simulink library "LopesDevelopmentLibrary"  (R2015b)
settings: Solver=ode45  StartTime=0.0  StopTime=10.0  RelTol=1e-3
values from neighbouring files (symbols this model uses):
  d2r = @(d) d*(pi/180)    [LopesDevelopmentLibrary_LoadParameters.m]
  ts = LopesParams.ts    [LopesDevelopmentLibrary_LoadParameters.m]
undefined symbols (not defined in the file or in its folder): anyParameterChanged, DiscIntNeverNeededParam, gcbh, LAP, LHF, LKF, LopesParams, macaddr, mxpcnetworkconfig, mxpcrtudprx, mxpcrtudptx, patientParametersChanged, port, PX, PZ, RAP, RHF, RKF, SelectorLOPESInSize, StrideTime_s, Time
undefined symbols (not defined in the file): LopesParamsSendDataArrayLen
libraries: LopesDevelopmentLibrary x327, simulink x100, dspmtrx3 x49, xpciplib x6, xpcnetworkbufferlib x5, dspsigops x4, dspstat3 x3, xpcethernetlib x2, visionstatistics x2, xpcseriallib x2, LopesDevelopmentLibraryTest x1, nmc x1
(part 7 of 12)

== system LopesDevelopmentLibrary/GaitPhaseDetection/Gait Phase Detection with Wrapper/No speed detection ==
  note: If COP is 5x closer to foot 1 than foot 2, foot 2 is assumed to be in swing
  note: Detection
      | 1 = stance phase
      | 2 = swing phase
  note: If the treadmill velocity is above 0.05 and 250 ms have passed
      | since the start of the simulation, gait initiation can be detected using the "normal" method
      | If Velocity of treadmill is too low, the COP is used to estimate swing/stance
  curVel : Inport
  CartesianPositions : Inport  Port=2
  Treadmill : Inport  Port=3
  "   " : MinMax
  "        " : simulink/Discrete/Tapped Delay  vinit=0  samptime=-1  NumDelays=250  DelayOrder=Oldest  includeCurrent=off
  Ankle_L_XZ : Selector  InputPortWidth=21  IndexOptions=Index vector (dialog)  Indices=[10 12]  OutputSizes=1
  Ankle_R_XZ : Selector  InputPortWidth=21  IndexOptions=Index vector (dialog)  Indices=[19 21]  OutputSizes=1
  COP_XZ : Selector  InputPortWidth=7  IndexOptions=Index vector (dialog)  Indices=[5 6]  OutputSizes=1
  Compare To Constant : simulink/Logic and Bit Operations/Compare To Constant  relop=<=  const=0.2  OutDataTypeStr=boolean
  Compare To Constant1 : simulink/Logic and Bit Operations/Compare To Constant  relop=>=  const=0.05  OutDataTypeStr=uint8  ZeroCross=off
  Compare To Constant2 : simulink/Logic and Bit Operations/Compare To Constant  relop=<=  const=0.2  OutDataTypeStr=boolean
  Constant : Constant  Value=2
  Constant1 : Constant
  Data Type Conversion : DataTypeConversion
  DistLeft : Fcn  Expr=((u(1) - u(3))^2 + (u(2) - u(4))^2)^0.5
  DistRight : Fcn  Expr=((u(1) - u(3))^2 + (u(2) - u(4))^2)^0.5
  Divide : Product  Inputs=*/
  Divide1 : Product  Inputs=*/
  LeftFoot : Switch  Criteria=u2 > Threshold
  Mux : Mux  Inputs=2
  Mux1 : Mux  Inputs=2
  RightFoot : Switch  Criteria=u2 > Threshold
  gaitSwitch : Outport
  Left : Outport  Port=2
  Right : Outport  Port=3
  wires:
  RightFoot/1 -> Right/1
  LeftFoot/1 -> Left/1
  Constant1/1 -> LeftFoot/3, RightFoot/3
  Constant/1 -> RightFoot/1, LeftFoot/1
  Compare To Constant2/1 -> LeftFoot/2
  Compare To Constant/1 -> RightFoot/2
  Divide1/1 -> Compare To Constant2/1
  Divide/1 -> Compare To Constant/1
  DistRight/1 -> Divide1/1, Divide/2
  DistLeft/1 -> Divide/1, Divide1/2
  Mux1/1 -> DistRight/1
  Ankle_R_XZ/1 -> Mux1/1
  COP_XZ/1 -> Mux/2, Mux1/2
  Ankle_L_XZ/1 -> Mux/1
  Mux/1 -> DistLeft/1
  Treadmill/1 -> COP_XZ/1
  CartesianPositions/1 -> Ankle_L_XZ/1, Ankle_R_XZ/1
  "   "/1 -> Compare To Constant1/1
  "        "/1 -> "   "/1
  Data Type Conversion/1 -> gaitSwitch/1
  curVel/1 -> "        "/1
  Compare To Constant1/1 -> Data Type Conversion/1

== system LopesDevelopmentLibrary/GaitPhaseDetection/Gait Phase Detection with Wrapper/Phase_selection ==
  LeftWalking : Inport
  RightWalking : Inport  Port=2
  Gait_switch : Inport  Port=3
  ankle_x_l : Inport  Port=4
  ankle_x_r : Inport  Port=5
  LeftStop : Inport  Port=6
  RightStop : Inport  Port=7
  Delay : Delay  DelayLength=1  InitialCondition=0
  MATLAB Function : MATLAB Function  TreatAsAtomicUnit=on
  Phase : Outport
  wires:
  RightStop/1 -> MATLAB Function/4(rightStop)
  LeftStop/1 -> MATLAB Function/3(leftStop)
  ankle_x_r/1 -> MATLAB Function/7(right_x)
  ankle_x_l/1 -> MATLAB Function/6(left_x)
  Gait_switch/1 -> MATLAB Function/5(switchSignal)
  RightWalking/1 -> MATLAB Function/2(rightWalking)
  LeftWalking/1 -> MATLAB Function/1(leftWalking)
  Delay/1 -> MATLAB Function/8(prev)
  MATLAB Function/1(y) -> Phase/1, Delay/1

== system LopesDevelopmentLibrary/GaitPhaseDetection/Gait Phase Detection with Wrapper/RightLegWalking ==
  note: Right foot detection
      | 1 = stance phase
      | 2 = swing phase
  ankle_y_r_dot : Inport
  ankle_x_r_dot : Inport  Port=2
  knee_angle_dot : Inport  Port=3
  belt_speed : Inport  Port=4
  Add2 : Sum  OutDataTypeStr=double
  Heel strike detection : Subsystem
  Heel strike_safety : Subsystem
  Logical Operator2 : Logic  Operator=OR  AllPortsSameDT=off  OutDataTypeStr=boolean
  Sample and Hold2 : dspsigops/Sample and Hold  trig=Rising edge  initCond=1  latchinput=off
  Toe-off detection : Subsystem
  right : Outport  OutDataTypeStr=double
  wires:
  knee_angle_dot/1 -> Toe-off detection/2(knee_angle_dot)
  Heel strike_safety/1(Heel_strike_safety) -> Logical Operator2/2
  belt_speed/1 -> Heel strike_safety/2(belt_speed)
  Toe-off detection/1(Toe_off) -> Add2/2
  Heel strike detection/1(Heel_strike) -> Logical Operator2/1
  ankle_y_r_dot/1 -> Heel strike detection/1(ankle_y_dot)  "ankle_y_dot"
  ankle_x_r_dot/1 -> Toe-off detection/1(ankle_x_dot), Heel strike detection/2(ankle_x_dot), Heel strike_safety/1(ankle_x_dot)  "ankle_x_dot"
  Add2/1 -> Sample and Hold2/1, Sample and Hold2/Trigger
  Logical Operator2/1 -> Add2/1
  Sample and Hold2/1 -> right/1

== system LopesDevelopmentLibrary/GaitPhaseDetection/Gait Phase Detection with Wrapper/Smart derivative ==
  note: The filter order is regulated by the belt speed to promote
      | efficiency and accuracy
  ankle_y_l : Inport
  ankle_x_l : Inport  Port=2
  angle_knee_l : Inport  Port=3
  ankle_y_r : Inport  Port=4
  ankle_x_r : Inport  Port=5
  angle_knee_r : Inport  Port=6
  treadmill speed : Inport  Port=7
  Filtered derivative : Subsystem
  Filtered derivative1 : Subsystem
  Filtered derivative2 : Subsystem
  Filtered derivative3 : Subsystem
  Filtered derivative4 : Subsystem
  Filtered derivative5 : Subsystem
  belt_speed to cut-off : Subsystem
  ankle_y_l_dot : Outport
  ankle_x_l_dot : Outport  Port=2
  angle_knee_l_dot : Outport  Port=3
  ankle_y_r_dot : Outport  Port=4
  ankle_x_r_dot : Outport  Port=5
  angle_knee_r_dot : Outport  Port=6
  wires:
  Filtered derivative1/1(x_dot) -> ankle_x_l_dot/1
  treadmill speed/1 -> belt_speed to cut-off/1(belt speed)
  belt_speed to cut-off/1(cut-off (hz)) -> Filtered derivative/2(cut-off (hz)), Filtered derivative1/2(cut-off (hz)), Filtered derivative2/2(cut-off (hz)), Filtered derivative3/2(cut-off (hz)), Filtered derivative4/2(cut-off (hz)), Filtered derivative5/2(cut-off (hz))
  Filtered derivative5/1(x_dot) -> angle_knee_r_dot/1
  Filtered derivative4/1(x_dot) -> ankle_x_r_dot/1
  Filtered derivative3/1(x_dot) -> ankle_y_r_dot/1
  Filtered derivative2/1(x_dot) -> angle_knee_l_dot/1
  angle_knee_r/1 -> Filtered derivative5/1(x)
  ankle_x_r/1 -> Filtered derivative4/1(x)
  ankle_y_r/1 -> Filtered derivative3/1(x)
  angle_knee_l/1 -> Filtered derivative2/1(x)
  ankle_x_l/1 -> Filtered derivative1/1(x)
  Filtered derivative/1(x_dot) -> ankle_y_l_dot/1
  ankle_y_l/1 -> Filtered derivative/1(x)

== system LopesDevelopmentLibrary/GaitPhaseDetection/Gait Phase detection/Data selection ==
  Cart_pos : Inport
  Treadmill : Inport  Port=2
  Angle_l : Subsystem
  Angle_r : Subsystem
  Selector : Selector  InputPortWidth=21  IndexOptions=Index vector (dialog)  Indices=[11]  OutputSizes=1
  Selector1 : Selector  InputPortWidth=21  IndexOptions=Index vector (dialog)  Indices=[20]  OutputSizes=1
  Selector10 : Selector  InputPortWidth=21  IndexOptions=Index vector (dialog)  Indices=[16 17 18]  OutputSizes=1
  Selector11 : Selector  InputPortWidth=21  IndexOptions=Index vector (dialog)  Indices=[13 14 15]  OutputSizes=1
  Selector2 : Selector  InputPortWidth=21  IndexOptions=Index vector (dialog)  Indices=[19]  OutputSizes=1
  Selector3 : Selector  InputPortWidth=21  IndexOptions=Index vector (dialog)  Indices=[10]  OutputSizes=1
  Selector4 : Selector  InputPortWidth=7  IndexOptions=Index vector (dialog)  Indices=[2]  OutputSizes=1
  Selector5 : Selector  InputPortWidth=21  IndexOptions=Index vector (dialog)  Indices=[10 11 12]  OutputSizes=1
  Selector6 : Selector  InputPortWidth=21  IndexOptions=Index vector (dialog)  Indices=[7 8 9]  OutputSizes=1
  Selector7 : Selector  InputPortWidth=21  IndexOptions=Index vector (dialog)  Indices=[4 5 6]  OutputSizes=1
  Selector9 : Selector  InputPortWidth=21  IndexOptions=Index vector (dialog)  Indices=[19 20 21]  OutputSizes=1
  ankle_y_l : Outport
  ankle_x_l : Outport  Port=2
  angle_knee_l : Outport  Port=3
  ankle_y_r : Outport  Port=4
  ankle_x_r : Outport  Port=5
  angle_knee_r : Outport  Port=6
  Treadmill speed : Outport  Port=7
  wires:
  Angle_r/1(angle_r) -> angle_knee_r/1
  Angle_l/1(angle_l) -> angle_knee_l/1
  Selector11/1 -> Angle_r/3(hip)
  Selector9/1 -> Angle_r/1(ankle)
  Selector10/1 -> Angle_r/2(knee)
  Selector7/1 -> Angle_l/3(hip)
  Selector6/1 -> Angle_l/2(knee)
  Selector5/1 -> Angle_l/1(ankle)
  Cart_pos/1 -> Selector/1, Selector3/1, Selector1/1, Selector2/1, Selector6/1, Selector7/1, Selector9/1, Selector11/1, Selector10/1, Selector5/1
  Selector/1 -> ankle_y_l/1
  Selector1/1 -> ankle_y_r/1
  Selector4/1 -> Treadmill speed/1
  Selector3/1 -> ankle_x_l/1
  Treadmill/1 -> Selector4/1
  Selector2/1 -> ankle_x_r/1

== system LopesDevelopmentLibrary/GaitPhaseDetection/Gait Phase detection/LeftLeg ==
  note: Left foot detection
      | 1 = stance phase
      | 2 = swing phase
  ankle_y_l_dot : Inport
  ankle_x_l_dot : Inport  Port=2
  knee_theta_l_dot : Inport  Port=3
  belt_speed : Inport  Port=4
  Add1 : Sum
  Heel strike detection : Subsystem
  Heel strike_safety : Subsystem
  Logical Operator1 : Logic  Operator=OR  AllPortsSameDT=off  OutDataTypeStr=boolean
  Sample and Hold1 : dspsigops/Sample and Hold  trig=Rising edge  initCond=1  latchinput=off
  Toe-off detection : Subsystem
  left : Outport
  wires:
  knee_theta_l_dot/1 -> Toe-off detection/2(knee_angle_dot)
  Heel strike_safety/1(Heel_strike_safety) -> Logical Operator1/2
  belt_speed/1 -> Heel strike_safety/2(belt_speed)
  Toe-off detection/1(Toe_off) -> Add1/2
  Heel strike detection/1(Heel_strike) -> Logical Operator1/1
  ankle_y_l_dot/1 -> Heel strike detection/1(ankle_y_dot)  "ankle_y_dot"
  ankle_x_l_dot/1 -> Heel strike detection/2(ankle_x_dot), Toe-off detection/1(ankle_x_dot), Heel strike_safety/1(ankle_x_dot)  "ankle_x_dot"
  Add1/1 -> Sample and Hold1/1, Sample and Hold1/Trigger
  Logical Operator1/1 -> Add1/1
  Sample and Hold1/1 -> left/1

== system LopesDevelopmentLibrary/GaitPhaseDetection/Gait Phase detection/No speed detection ==
  note: If the treadmill velocity is above 0.05 and 1.5 seconds have passed
      | since the start of the simulation, gait initiation can be detected
  curVel : Inport
  "   " : MinMax
  "        " : simulink/Discrete/Tapped Delay  vinit=0  samptime=-1  NumDelays=1500  DelayOrder=Oldest  includeCurrent=off
  Compare To Constant1 : simulink/Logic and Bit Operations/Compare To Constant  relop=>=  const=0.05  OutDataTypeStr=uint8  ZeroCross=off
  Data Type Conversion : DataTypeConversion
  gaitSwitch : Outport
  wires:
  "   "/1 -> Compare To Constant1/1
  "        "/1 -> "   "/1
  Data Type Conversion/1 -> gaitSwitch/1
  curVel/1 -> "        "/1
  Compare To Constant1/1 -> Data Type Conversion/1

== system LopesDevelopmentLibrary/GaitPhaseDetection/Gait Phase detection/Phase_selection ==
  Left : Inport
  Right : Inport  Port=2
  Gait_switch : Inport  Port=3
  ankle_x_l : Inport  Port=4
  ankle_x_r : Inport  Port=5
  MATLAB Function : MATLAB Function  TreatAsAtomicUnit=on
  Phase : Outport
  wires:
  ankle_x_r/1 -> MATLAB Function/5(right_x)
  ankle_x_l/1 -> MATLAB Function/4(left_x)
  Gait_switch/1 -> MATLAB Function/3(belt)
  Right/1 -> MATLAB Function/2(right)
  Left/1 -> MATLAB Function/1(left)
  MATLAB Function/1(y) -> Phase/1

== system LopesDevelopmentLibrary/GaitPhaseDetection/Gait Phase detection/RightLeg ==
  note: Right foot detection
      | 1 = stance phase
      | 2 = swing phase
  ankle_y_r_dot : Inport
  ankle_x_r_dot : Inport  Port=2
  knee_angle_dot : Inport  Port=3
  belt_speed : Inport  Port=4
  Add2 : Sum
  Heel strike detection1 : Subsystem
  Heel strike_safety1 : Subsystem
  Logical Operator2 : Logic  Operator=OR  AllPortsSameDT=off  OutDataTypeStr=boolean
  Sample and Hold2 : dspsigops/Sample and Hold  trig=Rising edge  initCond=1  latchinput=off
  Toe-off detection1 : Subsystem
  right : Outport
  wires:
  knee_angle_dot/1 -> Toe-off detection1/2(knee_angle_dot)
  Heel strike_safety1/1(Heel_strike_safety) -> Logical Operator2/2
  belt_speed/1 -> Heel strike_safety1/2(belt_speed)
  Toe-off detection1/1(Toe_off) -> Add2/2
  Heel strike detection1/1(Heel_strike) -> Logical Operator2/1
  ankle_y_r_dot/1 -> Heel strike detection1/1(ankle_y_dot)  "ankle_y_dot"
  ankle_x_r_dot/1 -> Heel strike_safety1/1(ankle_x_dot), Toe-off detection1/1(ankle_x_dot), Heel strike detection1/2(ankle_x_dot)  "ankle_x_dot"
  Add2/1 -> Sample and Hold2/1, Sample and Hold2/Trigger
  Logical Operator2/1 -> Add2/1
  Sample and Hold2/1 -> right/1

== system LopesDevelopmentLibrary/GaitPhaseDetection/Gait Phase detection/Smart derivative ==
  note: The filter order is regulated by the belt speed to promote
      | efficiency and accuracy
  ankle_y_l : Inport
  ankle_x_l : Inport  Port=2
  angle_knee_l : Inport  Port=3
  ankle_y_r : Inport  Port=4
  ankle_x_r : Inport  Port=5
  angle_knee_r : Inport  Port=6
  treadmill speed : Inport  Port=7
  Filtered derivative : Subsystem
  Filtered derivative1 : Subsystem
  Filtered derivative2 : Subsystem
  Filtered derivative3 : Subsystem
  Filtered derivative4 : Subsystem
  Filtered derivative5 : Subsystem
  belt_speed to cut-off : Subsystem
  ankle_y_l_dot : Outport
  ankle_x_l_dot : Outport  Port=2
  angle_knee_l_dot : Outport  Port=3
  ankle_y_r_dot : Outport  Port=4
  ankle_x_r_dot : Outport  Port=5
  angle_knee_r_dot : Outport  Port=6
  wires:
  Filtered derivative1/1(x_dot) -> ankle_x_l_dot/1
  treadmill speed/1 -> belt_speed to cut-off/1(belt speed)
  belt_speed to cut-off/1(cut-off (hz)) -> Filtered derivative5/2(cut-off (hz)), Filtered derivative4/2(cut-off (hz)), Filtered derivative3/2(cut-off (hz)), Filtered derivative2/2(cut-off (hz)), Filtered derivative1/2(cut-off (hz)), Filtered derivative/2(cut-off (hz))
  Filtered derivative5/1(x_dot) -> angle_knee_r_dot/1
  Filtered derivative4/1(x_dot) -> ankle_x_r_dot/1
  Filtered derivative3/1(x_dot) -> ankle_y_r_dot/1
  Filtered derivative2/1(x_dot) -> angle_knee_l_dot/1
  angle_knee_r/1 -> Filtered derivative5/1(x)
  ankle_x_r/1 -> Filtered derivative4/1(x)
  ankle_y_r/1 -> Filtered derivative3/1(x)
  angle_knee_l/1 -> Filtered derivative2/1(x)
  ankle_x_l/1 -> Filtered derivative1/1(x)
  Filtered derivative/1(x_dot) -> ankle_y_l_dot/1
  ankle_y_l/1 -> Filtered derivative/1(x)

== system LopesDevelopmentLibrary/Mindwalker/Mindwalker_Lopes_Conversion/CalculateForceOnTorso ==
  MW_SpringPositions : Inport
  MW_SpringVelocities : Inport  Port=2
  MW_SpringStiffness : Inport  Port=3
  MW_BiasForces : Inport  Port=4
  Lopes_ModelPos : Inport  Port=5
  Lopes_ModelVel : Inport  Port=6
  Inertia : Inport  Port=7
  Add : Sum  Inputs=1
  CalculateDampingTerm : Subsystem
  GetLHFandRHF : Selector  InputPortWidth=11  IndexOptions=Index vector (dialog)  Indices=[4,7]  OutputSizes=1
  GetLHFandRHF1 : Selector  InputPortWidth=8  IndexOptions=Index vector (dialog)  Indices=[4,7]  OutputSizes=1
  GetLHFandRHF2 : Selector  InputPortWidth=11  IndexOptions=Index vector (dialog)  Indices=[4,7]  OutputSizes=1
  GetLHFandRHF3 : Selector  InputPortWidth=8  IndexOptions=Index vector (dialog)  Indices=[4,7]  OutputSizes=1
  GetLHFandRHF4 : Selector  InputPortWidth=6  IndexOptions=Index vector (dialog)  Indices=[2,5]  OutputSizes=1
  GetLHFandRHF5 : Selector  InputPortWidth=6  IndexOptions=Index vector (dialog)  Indices=[2,5]  OutputSizes=1
  Mux : Mux  Inputs=3
  Product : Product  RndMeth=Zero
  Product1 : Product  RndMeth=Zero
  Subtract : Sum  Inputs=+-
  Subtract1 : Sum  Inputs=+-
  Unary Minus : UnaryMinus
  ForceOnTorso : Outport
  wires:
  Add/1 -> ForceOnTorso/1  "TotalForceOnTorso"
  MW_SpringVelocities/1 -> GetLHFandRHF3/1
  Inertia/1 -> CalculateDampingTerm/2(Inertia)
  MW_SpringStiffness/1 -> GetLHFandRHF4/1
  MW_BiasForces/1 -> GetLHFandRHF5/1
  Lopes_ModelPos/1 -> GetLHFandRHF/1
  MW_SpringPositions/1 -> GetLHFandRHF1/1
  GetLHFandRHF5/1 -> Unary Minus/1
  Unary Minus/1 -> Mux/3
  Mux/1 -> Add/1
  GetLHFandRHF3/1 -> Subtract1/1
  GetLHFandRHF2/1 -> Subtract1/2
  GetLHFandRHF1/1 -> Subtract/1
  GetLHFandRHF/1 -> Subtract/2
  CalculateDampingTerm/1(Damping) -> Product1/1
  Subtract/1 -> Product/2
  GetLHFandRHF4/1 -> CalculateDampingTerm/1(Stiffness), Product/1
  Subtract1/1 -> Product1/2
  Lopes_ModelVel/1 -> GetLHFandRHF2/1
  Product/1 -> Mux/1
  Product1/1 -> Mux/2

== system LopesDevelopmentLibrary/Mindwalker/Mindwalker_Lopes_Conversion/LopesToMWPosition ==
  note: This block works for angles as well as velocities
  note: Lopes_Joints:
      | PX (=0)
      | PZ (=0)
      | LHA
      | LHF (absolute; actually Left Thigh Angle)
      | LKF
      | RHA
      | RHF
      | RKF
      | ----
      | PY
      | PAX
      | POB
  note: MW_Joints:
      | LHA
      | LHFR (Left Hip Flexion, Relative)
      | LKF
      | RHA
      | RHFR (Right HIp Flexion, Relative)
      | RKF
      | -----
      | TF = TorsoFlexion (shouldes forward is positive)
      | TOB = TorsoObliquity (shoulders to right is positive)
  Lopes_Joints : Inport
  TorsoValue : Inport  Port=2
  Add : Sum
  Add1 : Sum
  Demux : Demux  Outputs=11
  Mux : Mux  Inputs=8
  Terminator{,1..4} (5 alike) : Terminator
  Zero : Constant  Value=0
  MW_Joints : Outport
  wires:
  Demux/7 -> Add1/1
  Add1/1 -> Mux/5  "RHFR"
  Demux/4 -> Add/1
  Add/1 -> Mux/2  "LHFR"
  Demux/11 -> Terminator4/1  "POB"
  Demux/10 -> Terminator3/1  "PAX"
  Demux/9 -> Terminator2/1  "PY"
  Zero/1 -> Mux/8  "TOB"
  Demux/8 -> Mux/6  "RKF"
  Demux/6 -> Mux/4  "RHA"
  Demux/5 -> Mux/3  "LKF"
  Demux/3 -> Mux/1  "LHA"
  Demux/2 -> Terminator1/1  "PZ"
  Demux/1 -> Terminator/1  "PX"
  TorsoValue/1 -> Mux/7, Add/2, Add1/2  "TF"
  Lopes_Joints/1 -> Demux/1
  Mux/1 -> MW_Joints/1

== system LopesDevelopmentLibrary/Mindwalker/Mindwalker_Lopes_Conversion/LopesToMWVelocity ==
  note: MW_Joints:
      | LHA
      | LHFR (Left Hip Flexion, Relative)
      | LKF
      | RHA
      | RHFR (Right HIp Flexion, Relative)
      | RKF
      | -----
      | TF = TorsoFlexion (shouldes forward is positive)
      | TOB = TorsoObliquity (shoulders to right is positive)
  note: Lopes_Joints:
      | PX (=0)
      | PZ (=0)
      | LHA
      | LHF (absolute; actually Left Thigh Angle)
      | LKF
      | RHA
      | RHF
      | RKF
      | ----
      | PY
      | PAX
      | POB
  note: This block works for angles as well as velocities
  Lopes_Joints : Inport
  TorsoValue : Inport  Port=2
  Add : Sum
  Add1 : Sum
  Demux : Demux  Outputs=11
  Mux : Mux  Inputs=8
  Terminator{,1..4} (5 alike) : Terminator
  Zero : Constant  Value=0
  MW_Joints : Outport
  wires:
  Mux/1 -> MW_Joints/1
  Lopes_Joints/1 -> Demux/1
  TorsoValue/1 -> Add1/2, Add/2, Mux/7  "TF"
  Demux/1 -> Terminator/1  "PX"
  Demux/2 -> Terminator1/1  "PZ"
  Demux/3 -> Mux/1  "LHA"
  Demux/5 -> Mux/3  "LKF"
  Demux/6 -> Mux/4  "RHA"
  Demux/8 -> Mux/6  "RKF"
  Zero/1 -> Mux/8  "TOB"
  Demux/9 -> Terminator2/1  "PY"
  Demux/10 -> Terminator3/1  "PAX"
  Demux/11 -> Terminator4/1  "POB"
  Add/1 -> Mux/2  "LHFR"
  Demux/4 -> Add/1
  Add1/1 -> Mux/5  "RHFR"
  Demux/7 -> Add1/1

== system LopesDevelopmentLibrary/Mindwalker/Mindwalker_Lopes_Conversion/MWToLopesPosition ==
  note: RelativeJoints:
      | LHA
      | LHFR (Left Hip Flexion, Relative)
      | LKF
      | RHA
      | RHFR (Right HIp Flexion, Relative)
      | RKF
  note: AbsoluteJoints:
      | PX (=0)
      | PZ (=0)
      | LHA
      | LHF (absolute; actually Left Thigh Angle)
      | LKF
      | RHA
      | RHF
      | RKF
  note: This block works for angles as well as velocities
  RelativeJoints : Inport
  TorsoValue : Inport  Port=2
  Demux : Demux  Outputs=6
  Mux : Mux  Inputs=8
  Subtract : Sum  Inputs=+-
  Subtract1 : Sum  Inputs=+-
  Zero : Constant  Value=0
  Zero1 : Constant  Value=0
  AbsoluteJoints : Outport
  wires:
  Demux/4 -> Mux/6  "RHA"
  Demux/3 -> Mux/5  "LKF"
  Mux/1 -> AbsoluteJoints/1
  Demux/6 -> Mux/8  "RKF"
  Zero/1 -> Mux/1  "PX"
  RelativeJoints/1 -> Demux/1
  Demux/2 -> Subtract/1
  Zero1/1 -> Mux/2  "PZ"
  Demux/1 -> Mux/3  "LHA"
  Subtract/1 -> Mux/4  "LHF"
  TorsoValue/1 -> Subtract1/2, Subtract/2
  Demux/5 -> Subtract1/1
  Subtract1/1 -> Mux/7  "RHF"

== system LopesDevelopmentLibrary/Mindwalker/Mindwalker_Lopes_Conversion/MWToLopesVelocity ==
  note: This block works for angles as well as velocities
  note: AbsoluteJoints:
      | PX (=0)
      | PZ (=0)
      | LHA
      | LHF (absolute; actually Left Thigh Angle)
      | LKF
      | RHA
      | RHF
      | RKF
  note: RelativeJoints:
      | LHA
      | LHFR (Left Hip Flexion, Relative)
      | LKF
      | RHA
      | RHFR (Right HIp Flexion, Relative)
      | RKF
  RelativeJoints : Inport
  TorsoValue : Inport  Port=2
  Demux : Demux  Outputs=6
  Mux : Mux  Inputs=8
  Subtract : Sum  Inputs=+-
  Subtract1 : Sum  Inputs=+-
  Zero : Constant  Value=0
  Zero1 : Constant  Value=0
  AbsoluteJoints : Outport
  wires:
  Subtract1/1 -> Mux/7  "RHF"
  Demux/5 -> Subtract1/1
  TorsoValue/1 -> Subtract/2, Subtract1/2
  Subtract/1 -> Mux/4  "LHF"
  Demux/1 -> Mux/3  "LHA"
  Zero1/1 -> Mux/2  "PZ"
  Demux/2 -> Subtract/1
  RelativeJoints/1 -> Demux/1
  Zero/1 -> Mux/1  "PX"
  Demux/6 -> Mux/8  "RKF"
  Mux/1 -> AbsoluteJoints/1
  Demux/3 -> Mux/5  "LKF"
  Demux/4 -> Mux/6  "RHA"

== system LopesDevelopmentLibrary/Mindwalker/Mindwalker_Lopes_Conversion/TorsoDynamics ==
  note: This block calculates the torso angle and velocity. Bending forward is positive.
      | The UnitDelay is to make sure we don't get algebraic loops.
  Force : Inport
  Inertia : Inport  Port=2
  Add : Sum
  CalcTorsoAcc : Product  Inputs=*/
  CalcTorsoFlexion : Integrator
  CalcTorsoVelocity : Integrator
  EndStops : Subsystem
  Sum : Sum  Inputs=|++
  TorsoSpring : Subsystem
  Unit Delay : UnitDelay  SampleTime=-1
  TorsoFlexion : Outport
  TorsoFlexionVelocity : Outport  Port=2
  wires:
  Add/1 -> Sum/2
  TorsoSpring/1(Force) -> Add/2
  EndStops/1(EndstopForce) -> Add/1
  Force/1 -> Sum/1
  CalcTorsoFlexion/1 -> TorsoSpring/1(TorsoPos), EndStops/1(TorsoPos), TorsoFlexion/1
  CalcTorsoVelocity/1 -> CalcTorsoFlexion/1, TorsoSpring/2(TorsoVel), EndStops/2(TorsoVel), TorsoFlexionVelocity/1
  Inertia/1 -> CalcTorsoAcc/2, EndStops/3(TorsoInertia), TorsoSpring/3(TorsoInertia)
  Sum/1 -> Unit Delay/1
  CalcTorsoAcc/1 -> CalcTorsoVelocity/1
  Unit Delay/1 -> CalcTorsoAcc/1

== system LopesDevelopmentLibrary/Mindwalker/Mindwalker_Lopes_Conversion/VisualizeStickFigure ==
  TorsoFlexion : Inport
  Lopes_ModelPos : Inport  Port=2
  Enable : Inport  Port=3
  GetActuatedJoints : Selector  InputPortWidth=11  IndexOptions=Index vector (dialog)  Indices=1:8  OutputSizes=1
  Mux3 : Mux  Inputs=2
  Rate Transition : RateTransition
  Subsystem : Subsystem
  wires:
  Enable/1 -> Subsystem/Enable
  Rate Transition/1 -> Subsystem/1(In1)
  GetActuatedJoints/1 -> Mux3/1
  Lopes_ModelPos/1 -> GetActuatedJoints/1
  TorsoFlexion/1 -> Mux3/2
  Mux3/1 -> Rate Transition/1

== system LopesDevelopmentLibrary/Robot control blocks/FromLopes/GenerateString ==
  EnableAnaloginput : Inport
  Enable : EnablePort
  FromLopes_GenerateString : S-Function  InitFcn=try, set_param(gcb,'FunctionName','FromLopes_GenerateString'), end  FunctionName=FromLopes_GenerateString  SFunctionModules=FromLopes_GenerateString_wrapper  SFunctionDeploymentMode=off  EnableBusSupport=off  mask(S-Function Builder){}
      mask help: Simulink:masks:SFunctionBuilder_MD
      mask init: same as LopesDevelopmentLibrary/Various/SLRTMessage/S-Function Builder
      settings: CopyFcn=set_param(gcbh,'LinkStatus','none')  PreSaveFcn=try, set_param(gcb,'FunctionName','FromLopes_GenerateString'), end  OpenFcn=sfunctionwizard(gcbh)
      mask Display: plot(val(:,1),val(:,2)),disp(sys), port_label('input',1,'EnableAnalogInput'), port_label('output',1,'s'), port_label('output',2,'s_len')
  s : Outport
  s_len : Outport  Port=2
  wires:
  EnableAnaloginput/1 -> FromLopes_GenerateString/1
  FromLopes_GenerateString/1 -> s/1
  FromLopes_GenerateString/2 -> s_len/1

== system LopesDevelopmentLibrary/Robot control blocks/FromLopes/ParseString ==
  In1 : Inport
  In2 : Inport  Port=2
  Enable : EnablePort
  Data Type Conversion : DataTypeConversion  OutDataTypeStr=double
  FromLopes_ParseString : S-Function  InitFcn=try, set_param(gcb,'FunctionName','FromLopes_ParseString'), end  FunctionName=FromLopes_ParseString  SFunctionModules=FromLopes_ParseString_wrapper  SFunctionDeploymentMode=off  EnableBusSupport=off  mask(S-Function Builder){}
      mask help: Simulink:masks:SFunctionBuilder_MD
      mask init: same as LopesDevelopmentLibrary/Various/SLRTMessage/S-Function Builder
      settings: CopyFcn=set_param(gcbh,'LinkStatus','none')  PreSaveFcn=try, set_param(gcb,'FunctionName','FromLopes_ParseString'), end  OpenFcn=sfunctionwizard(gcbh)
      mask Display: plot(val(:,1),val(:,2)),disp(sys), port_label('input',1,'str'), port_label('input',2,'len'), port_label('output',1,'msgId'), port_label('output',2,'cnt'), port_label('output',3,'cntExpected'), port_label('output',4,'segmentModelPos'), port_label('output',5,'segmentModelVel'), port_label('output',6,'segmentModelAcc'), port_label('output',7,'segmentMeasPos'), port_label('output',8,'segmentMeasForce'), port_label('output',9,'cartesianModelPos'), port_label('output',10,'treadmill'), port_label('output',11,'analogInput')
  Logical Operator : Logic  Inputs=1  AllPortsSameDT=off  OutDataTypeStr=boolean
  MeasuredSegmentToAnatomicAngles : Subsystem
  MeasuredSegmentToAnatomicAngles1 : Subsystem
  MeasuredSegmentToAnatomicAngles2 : Subsystem
  MeasuredSegmentToAnatomicAngles3 : Subsystem
  MeasuredSegmentToAnatomicForce : Subsystem
  Relational Operator : RelationalOperator  Operator=~=  OutDataTypeStr=boolean
  Vector2CartesianPositionsBus : Subsystem
  cnt1 : Display  Commented=on
  cntExpected1 : Display  Commented=on
  msgID : Display  Commented=on
  ~Debug : Subsystem
      mask Display: disp('')
  ParseError : Outport
  ModelPos : Outport  Port=2
  ModelVel : Outport  Port=3
  ModelAcc : Outport  Port=4
  MeasPos : Outport  Port=5
  MeasForce : Outport  Port=6
  ModelCartPos : Outport  Port=7
  Treadmill : Outport  Port=8
  AnalogInput : Outport  Port=9
  wires:
  Logical Operator/1 -> Data Type Conversion/1
  FromLopes_ParseString/11 -> AnalogInput/1
  Data Type Conversion/1 -> ParseError/1
  FromLopes_ParseString/3 -> Relational Operator/2, cntExpected1/1
  FromLopes_ParseString/2 -> Relational Operator/1, cnt1/1
  FromLopes_ParseString/1 -> msgID/1
  FromLopes_ParseString/9 -> Vector2CartesianPositionsBus/1(In)
  In1/1 -> FromLopes_ParseString/1
  MeasuredSegmentToAnatomicAngles/1(Anatomic) -> ModelPos/1
  MeasuredSegmentToAnatomicAngles1/1(Anatomic) -> ModelVel/1
  FromLopes_ParseString/10 -> Treadmill/1
  Relational Operator/1 -> Logical Operator/1
  FromLopes_ParseString/8 -> MeasuredSegmentToAnatomicForce/1(segmentMeasForce)
  In2/1 -> FromLopes_ParseString/2
  FromLopes_ParseString/6 -> MeasuredSegmentToAnatomicAngles2/1(segmentModelX)
  FromLopes_ParseString/4 -> MeasuredSegmentToAnatomicAngles/1(segmentModelX)
  FromLopes_ParseString/5 -> MeasuredSegmentToAnatomicAngles1/1(segmentModelX)
  FromLopes_ParseString/7 -> MeasuredSegmentToAnatomicAngles3/1(segmentModelX)
  MeasuredSegmentToAnatomicAngles3/1(Anatomic) -> MeasPos/1
  Vector2CartesianPositionsBus/1(CartesianPositions) -> ModelCartPos/1
  MeasuredSegmentToAnatomicAngles2/1(Anatomic) -> ModelAcc/1
  MeasuredSegmentToAnatomicForce/1(AnatomicForce) -> MeasForce/1

== system LopesDevelopmentLibrary/Robot control blocks/FromLopes/~Debug ==

== system LopesDevelopmentLibrary/Robot control blocks/GeneralLopes/AnyMessageWasReceived ==
  In1 : Inport
  Compare To Constant : simulink/Logic and Bit Operations/Compare To Constant  relop=~=  const=-1  OutDataTypeStr=boolean
  Ground : Ground
  S-R Flip-Flop : simulink_extras/Flip Flops/S-R Flip-Flop  initial_condition=0
  Terminator : Terminator
  Out1 : Outport
  wires:
  Ground/1 -> S-R Flip-Flop/2
  S-R Flip-Flop/2 -> Terminator/1
  Compare To Constant/1 -> S-R Flip-Flop/1
  In1/1 -> Compare To Constant/1
  S-R Flip-Flop/1 -> Out1/1

== system LopesDevelopmentLibrary/Robot control blocks/GeneralLopes/GenerateString ==
  note: It appears that the first 100 (approx) messages are not
      | received by the LLC (does it take time to init the network card?)
      | We do want to initially set some values. I tried to do that at the
      | first message sent, but as that is not received, that doesn't work.
      | So, we just check whether we have received any message; if so,
      | we send the initializing stuff. This is what the AnyMessageWasReceived..
      | is for.
  DesiredState : Inport
  SegmentInertia : Inport  Port=2
  WatchdogTimeout_ms : Inport  Port=3
  AnyMessageWasReceivedByLLC : Inport  Port=4
  Enable : EnablePort
  Compare To Constant : simulink/Logic and Bit Operations/Compare To Constant  relop===  const=8  OutDataTypeStr=boolean
  Counter Free-Running : simulink/Sources/Counter Free-Running  NumBits=16  tsamp=-1
  Data Type Conversion1 : DataTypeConversion  OutDataTypeStr=double
  Detect Change : simulink/Logic and Bit Operations/Detect Change  vinit=0  InputProcessing=Inherited  OutDataTypeStr=boolean
  Detect Change1 : simulink/Logic and Bit Operations/Detect Change  vinit=nan  InputProcessing=Inherited  OutDataTypeStr=boolean
  Detect Change3 : simulink/Logic and Bit Operations/Detect Change  vinit=0  InputProcessing=Inherited  OutDataTypeStr=boolean
  Gain : Gain  Gain=ones(8,1)
  GeneralLopes_GenerateString : S-Function  InitFcn=try, set_param(gcb,'FunctionName','GeneralLopes_GenerateString'), end  FunctionName=GeneralLopes_GenerateString  SFunctionModules=GeneralLopes_GenerateString_wrapper  SFunctionDeploymentMode=off  EnableBusSupport=off  mask(S-Function Builder){}
      mask help: Simulink:masks:SFunctionBuilder_MD
      mask init: same as LopesDevelopmentLibrary/Various/SLRTMessage/S-Function Builder
      settings: CopyFcn=set_param(gcbh,'LinkStatus','none')  PreSaveFcn=try, set_param(gcb,'FunctionName','GeneralLopes_GenerateString'), end  OpenFcn=sfunctionwizard(gcbh)
      mask Display: plot(val(:,1),val(:,2)),disp(sys), port_label('input',1,'DesiredState'), port_label('input',2,'DesiredStateChanged'), port_label('input',3,'SegmentInertia'), port_label('input',4,'SegmentInertiaChanged'), port_label('input',5,'WatchdogTimeout'), port_label('input',6,'i'), port_label('output',1,'s'), port_label('output',2,'s_len')
  IsFirstSample : LopesDevelopmentLibrary/Various/IsFirstSample
  Logical Operator : Logic  Operator=OR  Inputs=1  AllPortsSameDT=off  OutDataTypeStr=boolean
  Logical Operator1 : Logic  AllPortsSameDT=off  OutDataTypeStr=boolean
  Logical Operator2 : Logic  Operator=NOT  AllPortsSameDT=off  OutDataTypeStr=boolean
  Logical Operator3 : Logic  AllPortsSameDT=off  OutDataTypeStr=boolean
  Logical Operator5 : Logic  Operator=OR  AllPortsSameDT=off  OutDataTypeStr=boolean
  Rounding Function : Rounding
  Width : Width
  s : Outport
  s_len : Outport  Port=2
  wires:
  Rounding Function/1 -> GeneralLopes_GenerateString/1
  Logical Operator5/1 -> Logical Operator1/1
  Detect Change3/1 -> Logical Operator5/2
  AnyMessageWasReceivedByLLC/1 -> Detect Change3/1
  Data Type Conversion1/1 -> GeneralLopes_GenerateString/6
  Counter Free-Running/1 -> Data Type Conversion1/1
  Logical Operator2/1 -> Logical Operator3/1
  IsFirstSample/1 -> Logical Operator2/1
  Logical Operator3/1 -> GeneralLopes_GenerateString/2
  Logical Operator1/1 -> GeneralLopes_GenerateString/4
  Logical Operator/1 -> Logical Operator5/1
  Compare To Constant/1 -> Logical Operator1/2
  Width/1 -> Compare To Constant/1
  SegmentInertia/1 -> Gain/1, Width/1
  Gain/1 -> Detect Change1/1, GeneralLopes_GenerateString/3
  Detect Change1/1 -> Logical Operator/1
  Detect Change/1 -> Logical Operator3/2
  GeneralLopes_GenerateString/1 -> s/1
  DesiredState/1 -> Rounding Function/1, Detect Change/1
  GeneralLopes_GenerateString/2 -> s_len/1
  WatchdogTimeout_ms/1 -> GeneralLopes_GenerateString/5

== system LopesDevelopmentLibrary/Robot control blocks/GeneralLopes/ParseString ==
  s : Inport
  s_len : Inport  Port=2
  Enable : EnablePort
  GeneralLopes_ParseString : S-Function  InitFcn=try, set_param(gcb,'FunctionName','GeneralLopes_ParseString'), end  FunctionName=GeneralLopes_ParseString  SFunctionModules=GeneralLopes_ParseString_wrapper  SFunctionDeploymentMode=off  EnableBusSupport=off  mask(S-Function Builder){}
      mask help: Simulink:masks:SFunctionBuilder_MD
      mask init: same as LopesDevelopmentLibrary/Various/SLRTMessage/S-Function Builder
      settings: CopyFcn=set_param(gcbh,'LinkStatus','none')  PreSaveFcn=try, set_param(gcb,'FunctionName','GeneralLopes_ParseString'), end  OpenFcn=sfunctionwizard(gcbh)
      mask Display: plot(val(:,1),val(:,2)),disp(sys), port_label('input',1,'s'), port_label('input',2,'s_len'), port_label('output',1,'isParseException'), port_label('output',2,'llcState'), port_label('output',3,'blueCabinetButtonPressed'), port_label('output',4,'isInitOk'), port_label('output',5,'isMotorsOk'), port_label('output',6,'isTreadmillEmpty'), port_label('output',7,'isPatientDefined')
  isParseException : Outport  InitialOutput=[-1]
  llcState : Outport  Port=2
  isBlueCabinetButtonPressed : Outport  Port=3
  isInitOk : Outport  Port=4
  isMotorsOk : Outport  Port=5
  isTreadmillEmpty : Outport  Port=6
  isPatientDefined : Outport  Port=7
  wires:
  GeneralLopes_ParseString/7 -> isPatientDefined/1  "isPatientDefined"
  GeneralLopes_ParseString/3 -> isBlueCabinetButtonPressed/1  "isCabinetBlueButtonPressed"
  GeneralLopes_ParseString/2 -> llcState/1  "llcState"
  GeneralLopes_ParseString/6 -> isTreadmillEmpty/1  "isTreadmillEmpty"
  GeneralLopes_ParseString/4 -> isInitOk/1  "isInitOk"
  GeneralLopes_ParseString/5 -> isMotorsOk/1  "isMotorsOk"
  s_len/1 -> GeneralLopes_ParseString/2
  s/1 -> GeneralLopes_ParseString/1
  GeneralLopes_ParseString/1 -> isParseException/1

== system LopesDevelopmentLibrary/Robot control blocks/GeneralLopes/~Debug ==

== system LopesDevelopmentLibrary/Robot control blocks/ToLopes/CrossFade ==
  In1 : Inport
  In2 : Inport  Port=2
  AmountIn2 : Inport  Port=3
  Add : Sum  Inputs=+-
  Add1 : Sum
  One : Constant
  Product : Product  RndMeth=Zero
  Product1 : Product  RndMeth=Zero
  Saturation : Saturate  UpperLimit=1  LowerLimit=0
  Out : Outport
  wires:
  Add1/1 -> Out/1
  In2/1 -> Product/1
  Product1/1 -> Add1/1
  Product/1 -> Add1/2
  Add/1 -> Product1/2
  Saturation/1 -> Add/2, Product/2
  One/1 -> Add/1
  AmountIn2/1 -> Saturation/1
  In1/1 -> Product1/1

== system LopesDevelopmentLibrary/Robot control blocks/ToLopes/CrossFade1 ==
  In1 : Inport
  In2 : Inport  Port=2
  AmountIn2 : Inport  Port=3
  Add : Sum  Inputs=+-
  Add1 : Sum
  One : Constant
  Product : Product  RndMeth=Zero
  Product1 : Product  RndMeth=Zero
  Saturation : Saturate  UpperLimit=1  LowerLimit=0
  Out : Outport
  wires:
  In1/1 -> Product1/1
  AmountIn2/1 -> Saturation/1
  One/1 -> Add/1
  Saturation/1 -> Product/2, Add/2
  Add/1 -> Product1/2
  Product/1 -> Add1/2
  Product1/1 -> Add1/1
  In2/1 -> Product/1
  Add1/1 -> Out/1

== system LopesDevelopmentLibrary/Robot control blocks/ToLopes/GenerateString ==
  note: MaxForces is an array of maximum joint
      | torques and applies to SpringSpring
      | and BiasForceSpring separately.
  UpdateSpringPositions : Inport
  SpringPositions : Inport  Port=2
  SpringVelocities : Inport  Port=3
  SpringStiffnesses : Inport  Port=4
  BiasForces : Inport  Port=5
  MaxForces : Inport  Port=6
  EffectsShouldBeEnabled : Inport  Port=7
  ForceSendEnableEffects : Inport  Port=8
  TreadmillVelocity : Inport  Port=9
  CreateSpringspring : Inport  Port=10
  CreateBiasForceSpring : Inport  Port=11
  Enable : EnablePort
  Detect Change : simulink/Logic and Bit Operations/Detect Change  vinit=0  InputProcessing=Inherited  OutDataTypeStr=boolean
  Detect Change1 : simulink/Logic and Bit Operations/Detect Change  vinit=0  InputProcessing=Inherited  OutDataTypeStr=boolean
  Detect Increase : simulink/Logic and Bit Operations/Detect Increase  vinit=0.0  InputProcessing=Inherited  OutDataTypeStr=boolean
  ForceSendTreadmillVelocity : Constant  Value=false  OutDataTypeStr=boolean
      settings: OpenFcn=|
      | b = get_param(gcb,'value');
      | if (strcmp(b,'true')),
      |   set_param (gcb,'value','false');
      | else
      |   set_param(gcb,'value','true');
      | end;
  Or : Logic  Operator=OR  Inputs=1  AllPortsSameDT=off  OutDataTypeStr=boolean
  OrEnableEffects : Logic  Operator=OR  AllPortsSameDT=off  OutDataTypeStr=boolean
  OrTreadmill : Logic  Operator=OR  AllPortsSameDT=off  OutDataTypeStr=boolean
  ToLopes_GenerateString : S-Function  InitFcn=try, set_param(gcb,'FunctionName','ToLopes_GenerateString'), end  FunctionName=ToLopes_GenerateString  SFunctionModules=ToLopes_GenerateString_wrapper  SFunctionDeploymentMode=off  EnableBusSupport=off  mask(S-Function Builder){}
      mask help: Simulink:masks:SFunctionBuilder_MD
      mask init: same as LopesDevelopmentLibrary/Various/SLRTMessage/S-Function Builder
      settings: CopyFcn=set_param(gcbh,'LinkStatus','none')  PreSaveFcn=try, set_param(gcb,'FunctionName','ToLopes_GenerateString'), end  OpenFcn=sfunctionwizard(gcbh)
      mask Display: plot(val(:,1),val(:,2)),disp(sys), port_label('input',1,'UpdateSpringSpringPositions'), port_label('input',2,'SpringPositions'), port_label('input',3,'SpringVelocities'), port_label('input',4,'SpringStiffnesses'), port_label('input',5,'BiasForces'), port_label('input',6,'MaxForces'), port_label('input',7,'UpdateMaxForces'), port_label('input',8,'TreadmillVelocity'), port_label('input',9,'TreadmillVelocityChanged'), port_label('input',10,'CreateSpringSpring'), port_label('input',11,'CreateBiasForceSpring'), port_label('input',12,'EnableEffects'), port_label('output',1,'s'), port_label('output',2,'s_len')
  s : Outport
  s_len : Outport  Port=2
  wires:
  UpdateSpringPositions/1 -> ToLopes_GenerateString/1
  OrEnableEffects/1 -> ToLopes_GenerateString/12
  Detect Increase/1 -> OrEnableEffects/1
  EffectsShouldBeEnabled/1 -> Detect Increase/1
  ForceSendTreadmillVelocity/1 -> OrTreadmill/2
  OrTreadmill/1 -> ToLopes_GenerateString/9
  Detect Change1/1 -> OrTreadmill/1
  TreadmillVelocity/1 -> ToLopes_GenerateString/8, Detect Change1/1
  SpringVelocities/1 -> ToLopes_GenerateString/3
  Or/1 -> ToLopes_GenerateString/7
  Detect Change/1 -> Or/1
  MaxForces/1 -> ToLopes_GenerateString/6, Detect Change/1
  ForceSendEnableEffects/1 -> OrEnableEffects/2
  CreateSpringspring/1 -> ToLopes_GenerateString/10
  CreateBiasForceSpring/1 -> ToLopes_GenerateString/11
  SpringPositions/1 -> ToLopes_GenerateString/2
  SpringStiffnesses/1 -> ToLopes_GenerateString/4
  ToLopes_GenerateString/2 -> s_len/1
  ToLopes_GenerateString/1 -> s/1
  BiasForces/1 -> ToLopes_GenerateString/5

== system LopesDevelopmentLibrary/Robot control blocks/ToLopes/GenerateVelocities ==
  note: This block allows you to choose different sources for the
      | velocity component of the springspring. Normal behaviour
      | (when ForceVelocityMethod=-1) is that it will use the user-provided
      | velocity if that is an 8-element array, and it will
      | use numerical derivative of the position signal if it the velocity input
      | is a scalar (i.e., in order to use the numerical derivative, you just need to
      | give a scalar constant at the input).
  note: ForceVelocityMethod:
      | -1: Auto (use user-proved velocities if available; use numerical derivative otherwise)
      | 0: ERROR
      | 1: User velocities
      | 2. Numerical Derivatives
      | 3. Filtered numerical derivatives (tau=0.01 s)
      | 4. Zero velocity
  Positions : Inport
  Velocities : Inport  Port=2
  SignalWidth : Inport  Port=3
  ForceVelocityMethod : Inport  Port=4
  Demux : Demux
  MATLAB Function : MATLAB Function  TreatAsAtomicUnit=on
  Merge : Merge  Inputs=4
  UseNumericalDerivative : Subsystem  TreatAsAtomicUnit=on
  UseNumericalDerivativeFiltered : Subsystem  TreatAsAtomicUnit=on
  UseUserVelocity : Subsystem  TreatAsAtomicUnit=on
  UseZeros : Subsystem  TreatAsAtomicUnit=on
  v_out : Outport
  wires:
  Velocities/1 -> UseUserVelocity/1(Velocities_in)
  SignalWidth/1 -> MATLAB Function/1(signalWidth)
  Demux/1 -> UseUserVelocity/Enable
  Positions/1 -> UseNumericalDerivative/1(Positions), UseNumericalDerivativeFiltered/1(Positions)
  Demux/2 -> UseNumericalDerivative/Enable
  ForceVelocityMethod/1 -> MATLAB Function/2(forceType)
  MATLAB Function/1(ena) -> Demux/1
  Demux/4 -> UseZeros/Enable
  Demux/3 -> UseNumericalDerivativeFiltered/Enable
  UseNumericalDerivativeFiltered/1(Velocities) -> Merge/3
  UseZeros/1(Velocities) -> Merge/4
  UseNumericalDerivative/1(Velocities) -> Merge/2
  UseUserVelocity/1(Velocities) -> Merge/1
  Merge/1 -> v_out/1

== system LopesDevelopmentLibrary/Robot control blocks/ToLopes/ParseString ==
  s : Inport
  In2 : Inport  Port=2
  Enable : EnablePort
  ToLopes_ParseString : S-Function  InitFcn=try, set_param(gcb,'FunctionName','ToLopes_ParseString'), end  FunctionName=ToLopes_ParseString  SFunctionModules=ToLopes_ParseString_wrapper  SFunctionDeploymentMode=off  EnableBusSupport=off  mask(S-Function Builder){}
      mask help: Simulink:masks:SFunctionBuilder_MD
      mask init: same as LopesDevelopmentLibrary/Various/SLRTMessage/S-Function Builder
      settings: CopyFcn=set_param(gcbh,'LinkStatus','none')  PreSaveFcn=try, set_param(gcb,'FunctionName','ToLopes_ParseString'), end  OpenFcn=sfunctionwizard(gcbh)
      mask Display: plot(val(:,1),val(:,2)),disp(sys), port_label('input',1,'s'), port_label('input',2,'s_len'), port_label('output',1,'ErrorValue'), port_label('output',2,'SpringSpringDidntExist'), port_label('output',3,'BiasForceSpringDidntExist')
  Error : Outport
  SpringSpringDidntExist : Outport  Port=2
  BiasForceSpringDidntExist : Outport  Port=3
  wires:
  ToLopes_ParseString/3 -> BiasForceSpringDidntExist/1
  ToLopes_ParseString/2 -> SpringSpringDidntExist/1
  ToLopes_ParseString/1 -> Error/1
  s/1 -> ToLopes_ParseString/1
  In2/1 -> ToLopes_ParseString/2

== system LopesDevelopmentLibrary/Robot control blocks/ToLopes/SwitchVelocitiesOnly ==
  note: `
  note: This block contains the logic for
      | using 'velocity only' control.
      | You should ONLY use it if
      | you have analytical derivatives of your
      | positions. If you have analytical second derivatives
      | as well, it will be more accurate
      | (use the block Various|BetterSpringVelocities)
      |
      | NOTE: UseAnalyticalVelocityOnly is more accurate (i.e., better),
      | but only usable if you have correct derivatives.
  note: The UseAnalyticalVelocityOnly block does not work properly
      | and (thus) should not be used until it's fixed. Please use the positions-and-velocity
      | mode.
      |
      | (the reason this doesn't work: I'm comparing the DesiredSpringPos with the ModelPosIn,
      | but I should compare it to the ActualSpringPos. I don't read that from the LLC yet, and adding
      | this requires some testing. So it is not a 1-minute fix.) - GvO, 151215
  UseAnalVelOnly : Inport
  ModelPosIn : Inport  Port=2
  DesSprPos : Inport  Port=3
  DesSprVel : Inport  Port=4
  Logical Operator : Logic  Operator=NOT  AllPortsSameDT=off  OutDataTypeStr=boolean
  Merge : Merge
  Merge1 : Merge
  Merge2 : Merge
  UseAnalyticalVelocityOnly : Subsystem
  UsePositionsAndVelocities : Subsystem
  UpdateSpringPos : Outport
  SpringPositions : Outport  Port=2
  SpringVelocities : Outport  Port=3
  wires:
  Logical Operator/1 -> UsePositionsAndVelocities/Enable
  UseAnalVelOnly/1 -> UseAnalyticalVelocityOnly/Enable, Logical Operator/1
  DesSprVel/1 -> UsePositionsAndVelocities/2(DesSprVel), UseAnalyticalVelocityOnly/3(DesSprVel)
  DesSprPos/1 -> UsePositionsAndVelocities/1(DesSprPos), UseAnalyticalVelocityOnly/2(DesSprPos)
  ModelPosIn/1 -> UseAnalyticalVelocityOnly/1(ModelPosIn)
  UsePositionsAndVelocities/3(SpringVelocities) -> Merge2/2
  UseAnalyticalVelocityOnly/3(SpringVelocities) -> Merge2/1
  UsePositionsAndVelocities/2(SpringPositions) -> Merge1/2
  UseAnalyticalVelocityOnly/2(SpringPositions) -> Merge1/1
  UsePositionsAndVelocities/1(UpdateSpringPos) -> Merge/2
  UseAnalyticalVelocityOnly/1(UpdateSpringPos) -> Merge/1
  Merge1/1 -> SpringPositions/1
  Merge2/1 -> SpringVelocities/1
  Merge/1 -> UpdateSpringPos/1

== system LopesDevelopmentLibrary/Robot control blocks/ToLopes/~Debug ==

== system LopesDevelopmentLibrary/Robot control blocks/ToLopes/~EnableLogic ==

== system LopesDevelopmentLibrary/Various/GenerateSyncPulseFromPhase/DetectPhaseSignalReset ==
  note: This block detects the event of phase reset (i.e., when it
      | goes from (approximately) 100 to (approximately) 0.
      | It does this by checking whether there is a decrease of at
      | least 50% within one sample time.
  Phase : Inport
  Compare To Constant : simulink/Logic and Bit Operations/Compare To Constant  relop=<  const=-50  OutDataTypeStr=boolean
  Subtract : Sum  Inputs=+-
  Unit Delay : UnitDelay  SampleTime=-1
  PhaseReset : Outport
  wires:
  Phase/1 -> Subtract/1, Unit Delay/1
  Compare To Constant/1 -> PhaseReset/1
  Unit Delay/1 -> Subtract/2
  Subtract/1 -> Compare To Constant/1

== system LopesDevelopmentLibrary/Various/GenerateSyncPulseFromPhase/GenerateRandomValue ==
  note: Generate a uniform random number between Minimum and Maximum each
      | time Trigger rises.
  Maximum : Inport
  Minimum : Inport  Port=2
  Trigger : TriggerPort  PortDimensions=1
  Add : Sum
  Product : Product  RndMeth=Zero
  Subtract : Sum  Inputs=+-
  Uniform Random Number : UniformRandomNumber  Minimum=0  Seed=66
  Out : Outport  InitialOutput=0
  wires:
  Maximum/1 -> Subtract/1
  Uniform Random Number/1 -> Product/1
  Product/1 -> Add/1
  Subtract/1 -> Product/2
  Add/1 -> Out/1
  Minimum/1 -> Add/2, Subtract/2

== system LopesDevelopmentLibrary/BlocksForInternalUse/GaitGeneration/CalculateCartesianPositions/ConvertFromAnkleAnglesToFootAngles ==
  note: Input for s-function,
      | jointAngles:
      | PelvisPosX
      | PelvixPosY
      | PelvisPosZ
      | PelvisAxialAngle
      | PelvisFrontalAngle
      | LHA
      | LHF
      | LHEndorotatoin
      | LKF
      | LAEndorotation
      | LAP
      | LAInversion
      | RHA
      | RHF
      | RHEnorotation
      | RKF
      | RAEndorotation
      | RAP
      | RAInversion
  note: The S-function uses absolute angles for the ankle angle,
      | and I use relative angles (relative to the lower leg).
      | This part converts it. It would be better to use
      | the same thing in both software parts however.
      | (but as long as we don't actuate/measure the ankle
      | angle, it doesn't matter at all.
  In : Inport
  Demux1 : Demux  Outputs=13
  Mux1 : Mux  Inputs=19
  Sum2 : Sum  Inputs=|-++
  Sum3 : Sum  Inputs=|-++
  Zero{,1,3..5,7} (6 alike) : Constant  Value=0
  Out : Outport
  wires:
  Sum3/1 -> Mux1/18  "RAP"
  Sum2/1 -> Mux1/11  "LAP"
  Zero7/1 -> Mux1/19  "RAI"
  Demux1/10 -> Sum3/3  "RAP"
  Zero5/1 -> Mux1/17  "RAE"
  Demux1/9 -> Sum3/2, Mux1/16  "RKF"
  Zero4/1 -> Mux1/15  "RHE"
  Demux1/8 -> Sum3/1, Mux1/14  "RHF"
  Demux1/7 -> Mux1/13  "RHA"
  Zero3/1 -> Mux1/12  "LAI"
  Demux1/6 -> Sum2/3  "LAP"
  Zero1/1 -> Mux1/10  "LAE"
  Demux1/5 -> Sum2/2, Mux1/9  "LKF"
  Zero/1 -> Mux1/8  "LHE"
  Demux1/4 -> Mux1/7, Sum2/1  "LHF"
  Demux1/3 -> Mux1/6  "LHA"
  Demux1/13 -> Mux1/5  "POB"
  Demux1/12 -> Mux1/4  "PAX"
  Demux1/11 -> Mux1/2  "PY"
  Demux1/2 -> Mux1/3  "PZ"
  Demux1/1 -> Mux1/1  "PX"
  In/1 -> Demux1/1
  Mux1/1 -> Out/1

== system LopesDevelopmentLibrary/BlocksForInternalUse/GaitGeneration/CalculateCartesianPositions/ExtractPatientParameters ==
  Parameters : Inport
  Bus Selector : BusSelector  OutputSignals=Patient.Mass_kg,Patient.BodyLength_m,Patient.PelvisWidth_m,Patient.PelvisHeight_m,Patient.UpperLegLength_m,Patient.LowerLegLength_m,Patient.FootLength_m,Patient.FootHeight_m,patientParametersChanged
  Data Type Conversion : DataTypeConversion  OutDataTypeStr=double
  Mux : Mux  Inputs=12
  PatientDimensions : Outport
  DimensionsChanged : Outport  Port=2
  wires:
  Data Type Conversion/1 -> DimensionsChanged/1
  Bus Selector/8 -> Mux/11, Mux/12  "<FootHeight_m>"
  Bus Selector/2 -> Mux/2  "<BodyLength_m>"
  Bus Selector/5 -> Mux/6, Mux/5  "<UpperLegLength_m>"
  Bus Selector/3 -> Mux/3  "<PelvisWidth_m>"
  Bus Selector/1 -> Mux/1  "<Mass_kg>"
  Bus Selector/7 -> Mux/9, Mux/10  "<FootLength_m>"
  Bus Selector/9 -> Data Type Conversion/1  "<patientParametersChanged>"
  Mux/1 -> PatientDimensions/1
  Bus Selector/6 -> Mux/7, Mux/8  "<LowerLegLength_m>"
  Parameters/1 -> Bus Selector/1
  Bus Selector/4 -> Mux/4  "<PelvisHeight_m>"

== system LopesDevelopmentLibrary/BlocksForInternalUse/GaitGeneration/CalculateCartesianPositions/OmitAnklesAndToes ==
  In : Inport
  Demux1 : Demux  Outputs=11
  Mux1 : Mux  Inputs=7
  Terminator{,1..3} (4 alike) : Terminator
  Out : Outport
  wires:
  Mux1/1 -> Out/1
  Demux1/10 -> Terminator2/1  "RightHeel"
  Demux1/11 -> Terminator3/1  "RightToe"
  Demux1/6 -> Terminator1/1  "LeftToe"
  Demux1/5 -> Terminator/1  "LeftHeel"
  Demux1/7 -> Mux1/5  "RightHip"
  Demux1/9 -> Mux1/7  "RightAnkle"
  Demux1/1 -> Mux1/1  "Pelvis"
  Demux1/2 -> Mux1/2  "LeftHip"
  Demux1/4 -> Mux1/4  "LeftAnkle"
  Demux1/8 -> Mux1/6  "RightKnee"
  In/1 -> Demux1/1
  Demux1/3 -> Mux1/3  "LeftKnee"

== system LopesDevelopmentLibrary/BlocksForInternalUse/GaitGeneration/CalculateReferenceGait/ActuatedDOFs ==
